simulink model "efficiency_losses_volatge_regulation"  (R2014b)
settings: Solver=ode23tb  StartTime=0.0  StopTime=5  MaxStep=1e-4  RelTol=1e-3
libraries: powerlib x8, powerlib_meascontrol x4
settings Model: Creator=Amr Saleh  LastModifiedBy=Amr Saleh

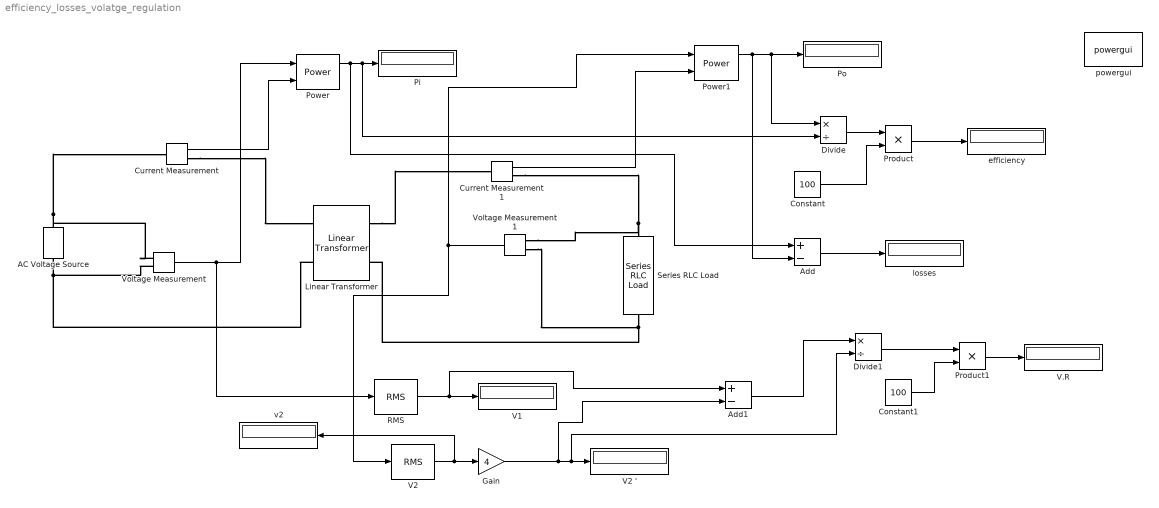
== system efficiency_losses_volatge_regulation ==
  AC Voltage Source : powerlib/Electrical Sources/AC Voltage Source  Amplitude=480*sqrt(2)  Phase=0  Frequency=50  SampleTime=0  Measurements=None
  Add : Sum  Inputs=+-
  Add1 : Sum  Inputs=+-
  Constant : Constant  Value=100
  Constant1 : Constant  Value=100
  Current Measurement : powerlib/Measurements/Current Measurement  PhasorSimulation=off  OutputType=Complex  PSBequivalent=0
  Current Measurement1 : powerlib/Measurements/Current Measurement  PhasorSimulation=off  OutputType=Complex  PSBequivalent=0
  Divide : Product  Inputs=*/
  Divide1 : Product  Inputs=*/
  Gain : Gain  Gain=4
  Linear Transformer : powerlib/Elements/Linear Transformer  UNITS=SI  NominalPower=[ 10000 50 ]  winding1=[480 0.6 3.183e-3]  winding2=[120 37.5e-3 1.989e-4]  ThreeWindings=off  winding3=[3.15e+05 0.7938 0.084225]  RmLm=[3000 1.591]  Measurements=None  DataType=on
  Pi : Display
  Po : Display
  Power : powerlib_meascontrol/Measurements/Power  Freq=50  Vinit=[1, 0]  Iinit=[1, 0]  Ts=0
  Power1 : powerlib_meascontrol/Measurements/Power  Freq=50  Vinit=[1, 0]  Iinit=[1, 0]  Ts=0
  Product : Product
  Product1 : Product
  RMS : powerlib_meascontrol/Measurements/RMS  TrueRMS=off  Freq=50  RMSInit=0  Ts=0
  Series RLC Load : powerlib/Elements/Series RLC Load  LConnTagsString=a  RConnTagsString=__new0  NominalVoltage=120  NominalFrequency=50  ActivePower=8500  InductivePower=5.267e3  CapacitivePower=0  Setx0=off  InitialVoltage=0  SetiL0=off  InitialCurrent=0  Measurements=None
  V.R : Display
  V1 : Display
  V2 : powerlib_meascontrol/Measurements/RMS  TrueRMS=off  Freq=50  RMSInit=0  Ts=0
  V2 ' : Display
  Voltage Measurement : powerlib/Measurements/Voltage Measurement  PhasorSimulation=off  OutputType=Complex  PSBequivalent=0
  Voltage Measurement1 : powerlib/Measurements/Voltage Measurement  PhasorSimulation=off  OutputType=Complex  PSBequivalent=0
  efficiency : Display
  losses : Display
  powergui : powerlib/powergui  Priority=1  SimulationMode=Continuous  SolverType=Tustin/Backward Euler (TBE)  SampleTime=50e-6  frequency=60  SPID=off  DisableSnubberDevices=off  DisableRonSwitches=off  DisableVfSwitches=off  SwTol=0  DisplayEquations=off  Interpol=off  methode=off  Ts=100  frequencyindice=50  Pbase=100e6  ErrMax=1e-4  Iterations=50  UnitsV=kV  UnitsW=MW  FunctionMessages=off  echomessages=off  HookPort=off  EnableUseOfTLC=off  x0status=blocks  RestoreLinks=warning  ResistiveCurrentMeasurement=off  Frange=[0:2:500]  Ylog=off  Xlog=on  ShowGrid=off  save=off  variable=ZData  structure=0  ZoomFFT=off  StartTime=0.0  cycles=1  DisplayStyle=1  fundamental=60  FreqAxis=off  MaxFrequency=1000  frequencyindicesteady=1  RmsSteady=1  display=off
  v2 : Display
  wires:
  Voltage Measurement/1 -> RMS/1, Power/1
  Current Measurement/1 -> Power/2
  Power/1 -> Add/1, Divide/2, Pi/1
  Voltage Measurement1/1 -> Power1/1, V2/1
  Current Measurement1/1 -> Power1/2
  Power1/1 -> Add/2, Divide/1, Po/1
  Divide/1 -> Product/1
  Constant/1 -> Product/2
  Product/1 -> efficiency/1
  Add/1 -> losses/1
  RMS/1 -> Add1/1, V1/1
  V2/1 -> v2/1, Gain/1
  Gain/1 -> Add1/2, Divide1/2, V2 '/1
  Add1/1 -> Divide1/1
  Divide1/1 -> Product1/1
  Constant1/1 -> Product1/2
  Product1/1 -> V.R/1
  connections:
  AC Voltage Source/RConn1 -- Current Measurement/LConn1 -- Voltage Measurement/LConn1
  Current Measurement/RConn1 -- Linear Transformer/LConn1
  Linear Transformer/LConn2 -- AC Voltage Source/LConn1 -- Voltage Measurement/LConn2
  Linear Transformer/RConn1 -- Current Measurement1/LConn1
  Current Measurement1/RConn1 -- Voltage Measurement1/LConn1 -- Series RLC Load/LConn1
  Series RLC Load/RConn1 -- Voltage Measurement1/LConn2 -- Linear Transformer/RConn2
